simulink model "position_control_ex"  (R2022b)
settings: Solver=ode4  StartTime=0.0  StopTime=300  FixedStep=0.01  RelTol=1e-3
model workspace (MAT data in the model file):
  mt = Simulink.Parameter
  mt.DataType = 'auto'
  mt.Complexity = 'real'
  mt.Dimensions = [0 0]
values from neighbouring files (symbols this model uses):
  m = 5000    [pid_variable.mat]
  m_d = 1.8    [pid_variable.mat]
libraries: slpidlib x1
settings Model: Creator=wlgns  LastModifiedBy=wlgns

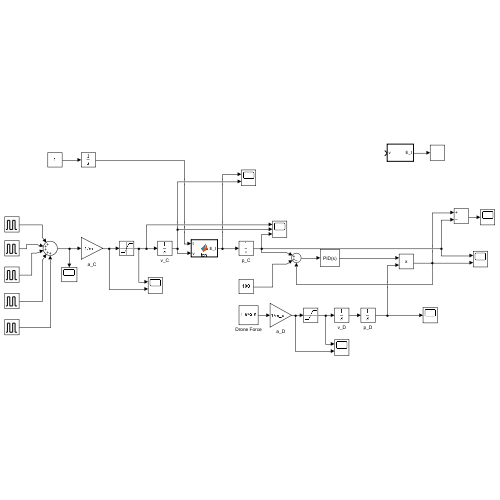
[thumbnail: Simulink's stored preview of the top-level diagram]
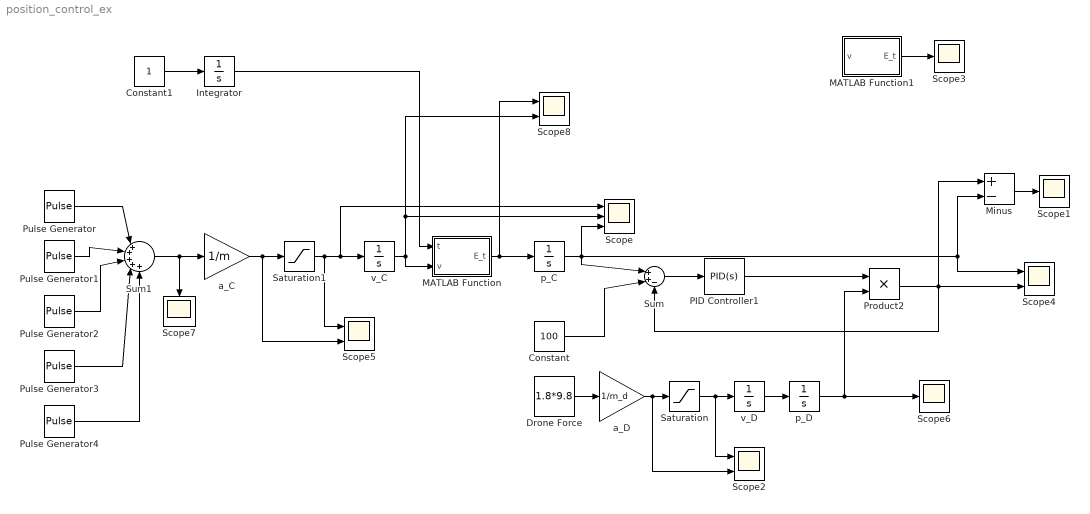
== system position_control_ex ==
  Constant : Constant  Value=100
  Constant1 : Constant
  Drone Force : Constant  Value=1.8*9.8
  Integrator : Integrator
  MATLAB Function : MATLAB Function  TreatAsAtomicUnit=on
  MATLAB Function1 : MATLAB Function  TreatAsAtomicUnit=on
  Minus : Sum  Inputs=+-
  PID Controller1 : slpidlib/PID Controller  Controller=PID  Form=Parallel  TimeDomain=Continuous-time  UseExternalTs=off  SampleTime=-1  IntegratorMethod=Forward Euler  FilterMethod=Forward Euler  ControllerParametersSource=internal  P=1.2  I=0.8  UseKiTs=off  D=0.5  N=100  UseFilter=on  TunerSelectOption=Transfer Function Based (PID Tuner App)  InitialConditionSource=internal  InitialConditionForIntegrator=0  InitialConditionForFilter=0  DifferentiatorICPrevScaledInput=0  ExternalReset=none  TrackingMode=off  Kt=1  LimitOutput=off  SatLimitsSource=internal  UpperSaturationLimit=inf  LowerSaturationLimit=-inf  LinearizeAsGain=on  AntiWindupMode=none  Kb=1  LimitIntegrator=off  UpperIntegratorSaturationLimit=inf  LowerIntegratorSaturationLimit=-inf  POutMin=[]  POutMax=[]  IOutMin=[]  IOutMax=[]  DOutMin=[]  DOutMax=[]  NOutMin=[]  NOutMax=[]  SumOutMin=[]  SumOutMax=[]  SaturationOutMin=[]  SaturationOutMax=[]  PParamMin=[]  PParamMax=[]  IParamMin=[]  IParamMax=[]  DParamMin=[]  DParamMax=[]  NParamMin=[]  NParamMax=[]  KbParamMin=[]  KbParamMax=[]  KtParamMin=[]  KtParamMax=[]  KbOutMin=[]  KbOutMax=[]  KtOutMin=[]  KtOutMax=[]  IntegratorOutMin=[]  IntegratorOutMax=[]  FilterOutMin=[]  FilterOutMax=[]  SumI1OutMin=[]  SumI1OutMax=[]  SumI2OutMin=[]  SumI2OutMax=[]  SumI3OutMin=[]  SumI3OutMax=[]  SumI4OutMin=[]  SumI4OutMax=[]  SumDOutMin=[]  SumDOutMax=[]  DifferentiatorOutMin=[]  DifferentiatorOutMax=[]  FilterDiffOutCoefMin=[]  FilterDiffOutCoefMax=[]  ReciprocalOutMin=[]  ReciprocalOutMax=[]  SumDenOutMin=[]  SumDenOutMax=[]  SumNumOutMin=[]  SumNumOutMax=[]  DivideOutMin=[]  DivideOutMax=[]  UdiffTsProdOutMin=[]  UdiffTsProdOutMax=[]  NTsProdOutMin=[]  NTsProdOutMax=[]  UintegralTsProdOutMin=[]  UintegralTsProdOutMax=[]  UngainTsProdOutMin=[]  UngainTsProdOutMax=[]  ClampingZeroOutDataTypeStr=Inherit: Inherit via back propagation  ClampingZeroOutMin=[]  ClampingZeroOutMax=[]  FilterDenConstantOutDataTypeStr=Inherit: Inherit via back propagation  FilterDenConstantOutMin=[]  FilterDenConstantOutMax=[]  PCopyOutDataTypeStr=Inherit: Inherit via back propagation  PCopyOutMin=[]  PCopyOutMax=[]  NCopyOutDataTypeStr=Inherit: Inherit via back propagation  NCopyOutMin=[]  NCopyOutMax=[]  IntegratorContinuousStateAttributes=''  IntegratorStateMustResolveToSignalObject=off  IntegratorRTWStateStorageClass=Auto  FilterContinuousStateAttributes=''  FilterStateMustResolveToSignalObject=off  FilterRTWStateStorageClass=Auto  ParallelPVariant=InternalParameters  IdealPVariant=Disabled  IVariant=InternalParameters  DVariant=InternalParameters  IntegratorVariant=Continuous  SatVariant=Disabled  AWVariant=Passthrough  PCopyVariant=Disabled  TRVariant=Disabled  FdbkBlocksVariant=Forward  IdealPFdbkVariant=Disabled  SatFdbkVariant=Disabled  DerivativeFilterVariant=ContFilter  NVariant=InternalParameters  NCopyVariant=Disabled  FilterICVariant=InternalICsFilter  IntegratorICVariant=InternalICs  ExternalResetVariant=Disabled  TRSumVariant=Passthrough  SumFdbkVariant=Disabled  SumVariant=Sum_PID  TsampFilterVariant=InternalTs  TsampNgainVariant=Passthrough  TsampIntegralVariant=Passthrough  ExternalSaturationOutDataTypeStr=Inherit: Same as second input
  Product2 : Product
  Pulse Generator : DiscretePulseGenerator  PulseType=Time based  Amplitude=30000  Period=17  PulseWidth=6  PhaseDelay=15
  Pulse Generator1 : DiscretePulseGenerator  PulseType=Time based  Amplitude=25000  Period=43  PulseWidth=8  PhaseDelay=35
  Pulse Generator2 : DiscretePulseGenerator  PulseType=Time based  Amplitude=15000  Period=23  PulseWidth=7  PhaseDelay=5
  Pulse Generator3 : DiscretePulseGenerator  PulseType=Time based  Amplitude=5000  Period=13  PulseWidth=30  PhaseDelay=5
  Pulse Generator4 : DiscretePulseGenerator  PulseType=Time based  Amplitude=10000  Period=53  PulseWidth=20  PhaseDelay=5
  Saturation : Saturate  UpperLimit=6  LowerLimit=0
  Saturation1 : Saturate  UpperLimit=6  LowerLimit=0  RndMeth=Nearest
  Scope : Scope  NumInputPorts=3
  Scope{1,3,6..7} (4 alike) : Scope
  Scope{2,4..5,8} (4 alike) : Scope  NumInputPorts=2
  Sum : Sum  Inputs=|++-
  Sum1 : Sum  Inputs=|+++++
  a_C : Gain  Gain=1/m
  a_D : Gain  Gain=1/m_d
  p_C : Integrator
  p_D : Integrator
  v_C : Integrator
  v_D : Integrator
  wires:
  v_C/1 -> Scope8/2, Scope/2, MATLAB Function/2(v)
  Sum/1 -> PID Controller1/1
  Constant/1 -> Sum/2
  p_C/1 -> Scope4/1, Minus/2, Sum/1, Scope/3
  Drone Force/1 -> a_D/1
  v_D/1 -> p_D/1
  p_D/1 -> Product2/2, Scope6/1
  Minus/1 -> Scope1/1
  PID Controller1/1 -> Product2/1
  a_D/1 -> Scope2/2, Saturation/1
  Saturation/1 -> Scope2/1, v_D/1
  Saturation1/1 -> Scope5/1, Scope/1, v_C/1
  Pulse Generator1/1 -> Sum1/2
  Sum1/1 -> Scope7/1, a_C/1
  Pulse Generator/1 -> Sum1/1
  Pulse Generator2/1 -> Sum1/3
  a_C/1 -> Scope5/2, Saturation1/1
  Pulse Generator3/1 -> Sum1/4
  Product2/1 -> Minus/1, Scope4/2, Sum/3
  MATLAB Function/1(E_t) -> Scope8/1, p_C/1
  Pulse Generator4/1 -> Sum1/5
  Constant1/1 -> Integrator/1
  MATLAB Function1/1(E_t) -> Scope3/1
  Integrator/1 -> MATLAB Function/1(t)

== matlab function position_control_ex/MATLAB Function1 ==
  settings: updateMethod=DISCRETE
  data: E_t output; v input
function E_t = fcn(v)
    persistent p_V;
    
    % 초기 호출 시 이전 속도 값을 초기화합니다.
    if isempty(p_V)
        p_V = 0;
    end
    
    % 30초마다 통신 오류가 발생하여 이전 1초 전의 속도 값을 가져옵니다.
    if mod(floor(v), 30) == 0
        E_t = p_V;
    else
        E_t = v;
    end
    
    % 이전 속도 값을 업데이트합니다.
    p_V = E_t;
end

== matlab function position_control_ex/MATLAB Function ==
  settings: updateMethod=DISCRETE
  data: t input; E_t output; v input
function E_t = fcn(t,v)
    persistent p_V;
    
    % 초기 호출 시 이전 속도 값을 초기화합니다.
    if isempty(p_V)
        p_V = 0;
    end
    
   % 30초마다 통신 오류가 발생하여 이전 1초 전의 속도 값을 가져옵니다.
    if mod(floor(t), 30) == 0
       E_t = p_V;
   else
      E_t = v;
    end
    
    %이전 속도 값을 업데이트합니다.
    p_V = E_t;
end
